simulink model "Stepper_Model_State_Feedback"  (R2017a)
settings: Solver=VariableStepAuto  StartTime=0.0  StopTime=60  RelTol=1e-3
undefined symbols (not defined in the file): K, Kz, Ptheta0, r, T, theta0
libraries: simulink x2
settings Model: Creator=Patrick  LastModifiedBy=Patrick

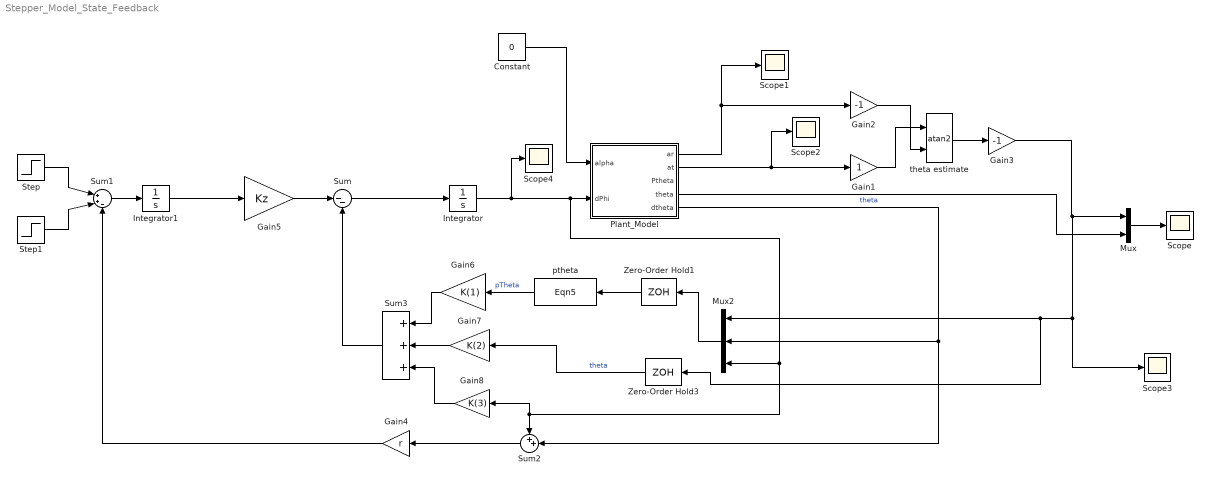
== system Stepper_Model_State_Feedback ==
  Constant : Constant  Value=0
  Gain1 : Gain
  Gain2 : Gain  Gain=-1
  Gain3 : Gain  Gain=-1
  Gain4 : Gain  Gain=r
  Gain5 : Gain  Gain=Kz
  Gain6 : Gain  Gain=K(1)
  Gain7 : Gain  Gain=K(2)
  Gain8 : Gain  Gain=K(3)
  Integrator : Integrator
  Integrator1 : Integrator
  Mux : Mux  Inputs=2
  Mux2 : Mux  Inputs=3
  Plant_Model : Subsystem
  Scope{,1..4} (5 alike) : Scope
  Step : Step  Time=10  After=.8  SampleTime=0
  Step1 : Step  Time=20  After=-.8*0  SampleTime=0
  Sum : Sum  Inputs=|--
  Sum1 : Sum  Inputs=|++-
  Sum2 : Sum  Inputs=++|
  Sum3 : Sum  Inputs=+++
  Zero-Order Hold1 : ZeroOrderHold  SampleTime=T
  Zero-Order Hold3 : ZeroOrderHold  SampleTime=T
  ptheta : MATLABFcn  MATLABFcn=Eqn5  OutputDimensions=[1 1]  Output1D=off
  theta estimate : Trigonometry  Operator=atan2  OutputSignalType=real
  wires:
  Constant/1 -> Plant_Model/1("alpha ")
  Mux/1 -> Scope/1
  Plant_Model/4(theta) -> Mux/2  "theta"
  Plant_Model/1(ar) -> Gain2/1, Scope1/1
  Plant_Model/2(at) -> Scope2/1, Gain1/1
  Gain1/1 -> theta estimate/1
  Gain2/1 -> theta estimate/2
  Integrator/1 -> Scope4/1, Plant_Model/2(dPhi), Mux2/3, Sum2/1, Gain8/1
  theta estimate/1 -> Gain3/1
  Gain3/1 -> Scope3/1, Zero-Order Hold3/1, Mux2/1, Mux/1
  Plant_Model/5(dtheta) -> Sum2/2, Mux2/2
  Zero-Order Hold1/1 -> ptheta/1
  Mux2/1 -> Zero-Order Hold1/1
  Zero-Order Hold3/1 -> Gain7/1  "theta"
  Sum/1 -> Integrator/1
  Sum3/1 -> Sum/2
  Sum1/1 -> Integrator1/1
  Sum2/1 -> Gain4/1
  Step/1 -> Sum1/1
  Gain5/1 -> Sum/1
  Integrator1/1 -> Gain5/1
  Gain4/1 -> Sum1/3
  Step1/1 -> Sum1/2
  ptheta/1 -> Gain6/1  "pTheta"
  Gain6/1 -> Sum3/1
  Gain7/1 -> Sum3/2
  Gain8/1 -> Sum3/3

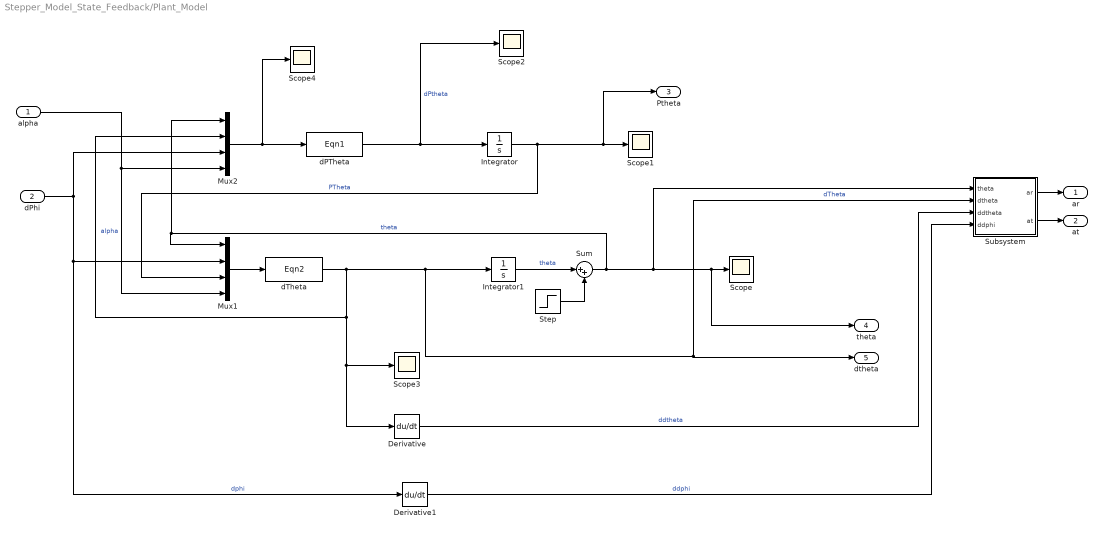
== system Stepper_Model_State_Feedback/Plant_Model ==
  "alpha " : Inport
  dPhi : Inport  Port=2
  Derivative : Derivative
  Derivative1 : Derivative
  Integrator : Integrator  InitialCondition=Ptheta0
  Integrator1 : Integrator  InitialCondition=theta0
  Mux1 : Mux  Inputs=[1 1 1 1]
  Mux2 : Mux  Inputs=[1 1 1 1]
  Scope{,1..4} (5 alike) : Scope
  Step : Step  Time=10  After=0  SampleTime=0
  Subsystem : Subsystem
  Sum : Sum  Inputs=|++
  dPTheta : MATLABFcn  MATLABFcn=Eqn1  OutputDimensions=[1 1]  Output1D=off
  dTheta : MATLABFcn  MATLABFcn=Eqn2  OutputDimensions=[1 1]  Output1D=off
  ar : Outport  PortDimensions=[1 1]
  at : Outport  Port=2  PortDimensions=[1 1]
  Ptheta : Outport  Port=3  PortDimensions=[1 1]
  theta : Outport  Port=4  PortDimensions=[1 1]
  dtheta : Outport  Port=5  PortDimensions=[1 1]
  wires:
  Integrator/1 -> Ptheta/1, Scope1/1, Mux1/3  "PTheta"
  dPhi/1 -> Mux2/3, Derivative1/1, Mux1/2  "dphi"
  dPTheta/1 -> Integrator/1, Scope2/1  "dPtheta"
  dTheta/1 -> Derivative/1, Scope3/1, Mux2/2, Subsystem/2(dtheta), dtheta/1, Integrator1/1  "dTheta"
  Mux2/1 -> Scope4/1, dPTheta/1
  Mux1/1 -> dTheta/1
  "alpha "/1 -> Mux1/4, Mux2/4  "alpha"
  Derivative/1 -> Subsystem/3(ddtheta)  "ddtheta"
  Derivative1/1 -> Subsystem/4(ddphi)  "ddphi"
  Subsystem/1(ar) -> ar/1
  Subsystem/2(at) -> at/1
  Sum/1 -> Mux1/1, Mux2/1, theta/1, Scope/1, Subsystem/1(theta)  "theta"
  Integrator1/1 -> Sum/1  "theta"
  Step/1 -> Sum/2

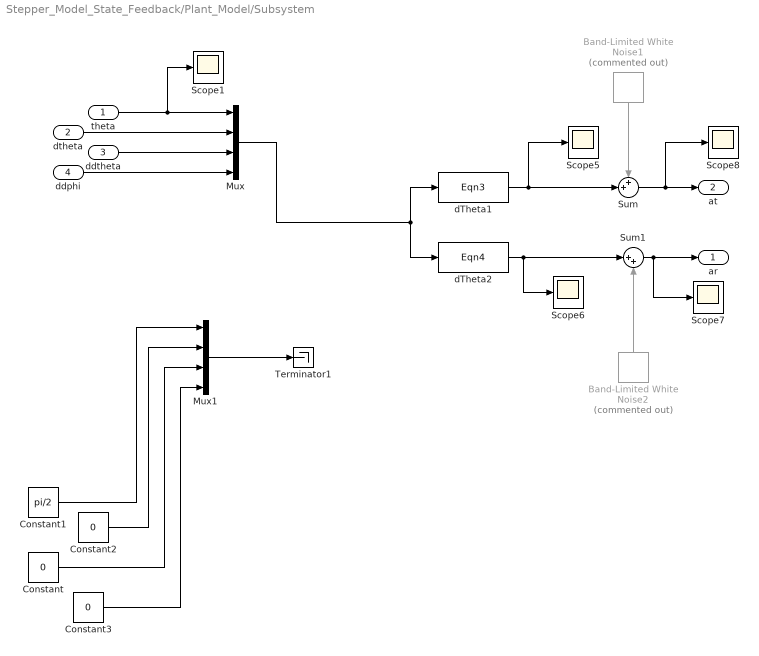
== system Stepper_Model_State_Feedback/Plant_Model/Subsystem ==
  theta : Inport
  dtheta : Inport  Port=2
  ddtheta : Inport  Port=3
  ddphi : Inport  Port=4
  Band-Limited White Noise1 : simulink/Sources/Band-Limited White Noise  Commented=on  Cov=[0.00001]  Ts=.01  seed=[23341]
  Band-Limited White Noise2 : simulink/Sources/Band-Limited White Noise  Commented=on  Cov=[0.00001]  Ts=.01  seed=[23341]
  Constant : Constant  Value=0
  Constant1 : Constant  Value=pi/2
  Constant2 : Constant  Value=0
  Constant3 : Constant  Value=0
  Mux : Mux
  Mux1 : Mux
  Scope{1,5..8} (5 alike) : Scope
  Sum : Sum  Inputs=++|
  Sum1 : Sum  Inputs=|++
  Terminator1 : Terminator
  dTheta1 : MATLABFcn  MATLABFcn=Eqn3  OutputDimensions=[1 1]  Output1D=off
  dTheta2 : MATLABFcn  MATLABFcn=Eqn4  OutputDimensions=[1 1]  Output1D=off
  ar : Outport  PortDimensions=[1 1]
  at : Outport  Port=2  PortDimensions=[1 1]
  wires:
  theta/1 -> Scope1/1, Mux/1
  dtheta/1 -> Mux/2
  Mux/1 -> dTheta1/1, dTheta2/1
  Sum/1 -> at/1, Scope8/1
  dTheta2/1 -> Sum1/1, Scope6/1
  Sum1/1 -> ar/1, Scope7/1
  dTheta1/1 -> Sum/2, Scope5/1
  ddphi/1 -> Mux/4
  ddtheta/1 -> Mux/3
  Band-Limited White Noise1/1 -> Sum/1
  Band-Limited White Noise2/1 -> Sum1/2
  Constant3/1 -> Mux1/4
  Constant1/1 -> Mux1/1
  Constant2/1 -> Mux1/2
  Constant/1 -> Mux1/3
  Mux1/1 -> Terminator1/1
